simulink model "SysModel"  (R2018a)
settings: Solver=VariableStepAuto  StartTime=0.0  StopTime=10.0  RelTol=1e-3
values from neighbouring files (symbols this model uses):
  A = [0      1              0           0 ... (first row only)    [PendulumSSModel.m]    (also in PendulumSSModel_LQR.m = [0                 1                 0                 0; PendulumSSModel_Metric.m = [0                 1                 0                 0; PendulumSSModel_Metric_fxn.m = [0                 1                 0                 0)
  B = [     0 ... (first row only)    [PendulumSSModel.m]    (also in PendulumSSModel_LQR.m = [        0; PendulumSSModel_Metric.m; PendulumSSModel_Metric_fxn.m)
  convFact = (100*Nom_V*Wheel_R*16)/(v*Stall_T)    (= 114.285714286)    [Pendulum_LQR.m]
  ic = [i_x, 0, i_phi, 0]'    [Pendulum_LQR.m]
  K = lqr(A,B,Q,R)    [PendulumSSModel_LQR.m]
  maxSig = 145    [Pendulum_LQR.m]
settings Model: Creator=jcl54  LastModifiedBy=jcl54

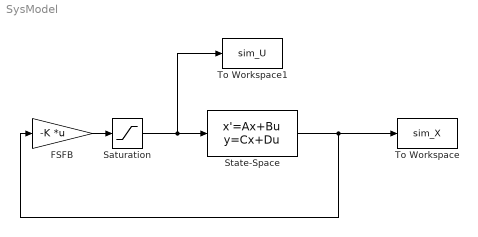
== system SysModel ==
  FSFB : Gain  Gain=-K  Multiplication=Matrix(K*u)
  Saturation : Saturate  UpperLimit=maxSig/convFact  LowerLimit=-maxSig/convFact
  State-Space : StateSpace  A=A  B=B  C=eye(4)  D=zeros(4,1)  InitialCondition=ic
  To Workspace : ToWorkspace  VariableName=sim_X  SaveFormat=Structure With Time  SampleTime=-1
  To Workspace1 : ToWorkspace  VariableName=sim_U  SaveFormat=Structure With Time  SampleTime=-1
  wires:
  State-Space/1 -> FSFB/1, To Workspace/1
  FSFB/1 -> Saturation/1
  Saturation/1 -> State-Space/1, To Workspace1/1
